simulink model "observermodel_final"  (R2020a)
settings: Solver=VariableStepAuto  StartTime=0.0  StopTime=U1(end,1)  RelTol=1e-3
values from neighbouring files (symbols this model uses):
  A = sys.A    [lqr_whitebox.m]    (also in lqr_whitebox.mat = [-0.00839310397514 0.00297468629139 0.0409151909921 -1.65614; matrices.mat = [-0.00839310397514 0.00297468629139 0.0409151909921 0 0.0029; model.m = 0.0009; pole_place_eef.m = A)
  B = sys.B    [lqr_whitebox.m]    (also in lqr_whitebox.mat = [0.00436783590621  1.30056082857e-18; -4.3352027619e-19  0.0; matrices.mat = [0.0043678359062  0; 0  0.0030268336543; 0  0; 0  0]; pole_place_eef.m = B; pole_placement.m)
  C = Ad.C    [Observer_mat.m]    (also in discretemodel.mat = [0  0  1  0; 0  0  0  1]; lqr_whitebox.m = sys.C; lqr_whitebox.mat = [0  0  1  0; 0  0  0  1]; matrices.mat = [0  0  1  0; 0  0  0  1])
  h = tout(2)-tout(1)    [Linearize_whitebox.m]    (also in Linearize_whitebox_final.m; Observer_mat.m; lqr_whitebox.mat = 1.00037043897; matrices.mat = 1.00080032013)
  K = [0.871464143609  0.0262786205748; 0.0262786205748  0.871464143609; 0.341518856741  0.00295216925623; 0.00295216925623  0.341518856741]    [K_matrix.mat]    (also in K_matrix_final.mat = [0.182524492646  0.00647209882564; 0.00436814029339  0.21194; Observer_mat.m = place(phi.',C.',P).'; lqr_whitebox.m = lqr(A,B,Q,R); lqr_whitebox.mat = [9.8403850338  0.823629600444  7.09136571585  0.104667034235)
settings Model: Creator=SIDTUDelft1  LastModifiedBy=SIDTUDelft1
settings DataIOCC: ReturnWorkspaceOutputs=off

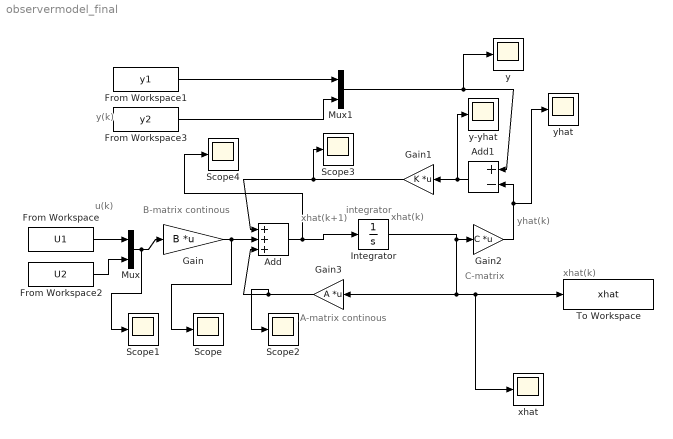
== system observermodel_final ==
  note: C-matrix
  note: integrator
  note: A-matrix continous
  note: B-matrix continous
  note: xhat(k)
  note: yhat(k)
  note: xhat(k)
  note: xhat(k+1)
  note: u(k)
  note: y(k)
  Add : Sum  Inputs=+++
  Add1 : Sum  Inputs=+-
  From Workspace : FromWorkspace  VariableName=U1  SampleTime=h
  From Workspace1 : FromWorkspace  VariableName=y1  SampleTime=h
  From Workspace2 : FromWorkspace  VariableName=U2  SampleTime=h
  From Workspace3 : FromWorkspace  VariableName=y2  SampleTime=h
  Gain : Gain  Gain=B  Multiplication=Matrix(K*u) (u vector)
  Gain1 : Gain  Gain=K  Multiplication=Matrix(K*u) (u vector)
  Gain2 : Gain  Gain=C  Multiplication=Matrix(K*u) (u vector)
  Gain3 : Gain  Gain=A  Multiplication=Matrix(K*u) (u vector)
  Integrator : Integrator  InitialCondition=290
  Mux : Mux  Inputs=2
  Mux1 : Mux  Inputs=2
  Scope{,1..4} (5 alike) : Scope
  To Workspace : ToWorkspace  VariableName=xhat  SampleTime=h
  xhat : Scope
  y : Scope
  y-yhat : Scope
  yhat : Scope
  wires:
  Gain/1 -> Scope/1, Add/2
  Add1/1 -> y-yhat/1, Gain1/1
  Gain1/1 -> Scope3/1, Add/1
  Add/1 -> Scope4/1, Integrator/1
  Gain2/1 -> yhat/1, Add1/2
  Gain3/1 -> Scope2/1, Add/3
  From Workspace/1 -> Mux/1
  From Workspace2/1 -> Mux/2
  Mux/1 -> Gain/1, Scope1/1
  From Workspace3/1 -> Mux1/2
  Mux1/1 -> y/1, Add1/1
  From Workspace1/1 -> Mux1/1
  Integrator/1 -> Gain3/1, xhat/1, To Workspace/1, Gain2/1
